simulink model "lab5starter"  (R2022b)
settings: Solver=FixedStepAuto  StartTime=0.0  StopTime=inf  FixedStep=0.002  RelTol=1e-3  EnableMultiTasking=on
undefined symbols (not defined in the file): HIL, Kc, qc_get_step_size, wf, z
libraries: quarc_library x4
settings Model: ExtModeTrigDuration=10000  Creator=lis3  LastModifiedBy=robert
settings SolverCC: PositivePriorityOrder=on
settings DebuggingCC: UnconnectedInputMsg=warning  UnconnectedOutputMsg=warning  UnconnectedLineMsg=warning
settings HardwareCC: ProdBitPerPointer=32  ProdBitPerSizeT=32  ProdBitPerPtrDiffT=32  ProdLargestAtomicInteger=Long  ProdWordSize=32  ProdHWDeviceType=ARM Compatible->ARM 7
settings ModelReferenceCC: EnableRefExpFcnMdlSchedulingChecks=on
settings RTWCC: Description=QUARC Linux RT ARMv7 Target (NI ELVIS III, NI myRIO) Using Toolchain  SystemTargetFile=quarc_linux_rt_armv7.tlc  Toolchain=QUARC linux_rt_armv7 | gmake (64-bit Windows)  BuildConfiguration=Faster Runs  DLArmComputeVersion=19.05
settings STFCustomTargetCC: TargetLangStandard=C99 (ISO)  ConcurrentExecutionCompliant=on  GRTInterface=on  UseToolchainInfoCompliant=on  SystemTargetFile=quarc_linux_rt_armv7.tlc
settings GRTTargetCC: ParMdlRefBuildCompliant=off  CompOptLevelCompliant=off  CombineOutputUpdateFcns=off  MatFileLogging=off  CPPClassGenCompliant=off  GRTInterface=on  ExtMode=on  ExtModeMexFile=quarc_comm  ExtModeMexArgs='-w -d /tmp -uri %u'

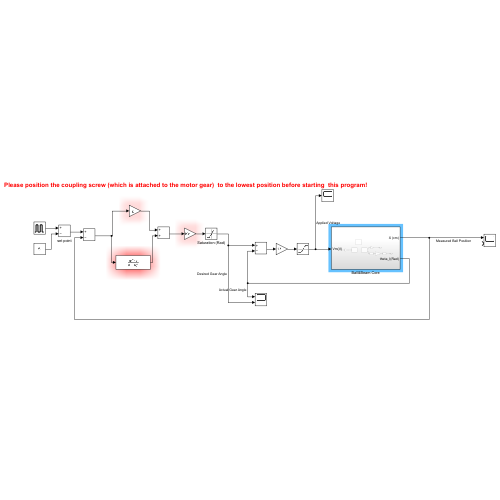
[thumbnail: Simulink's stored preview of the top-level diagram]
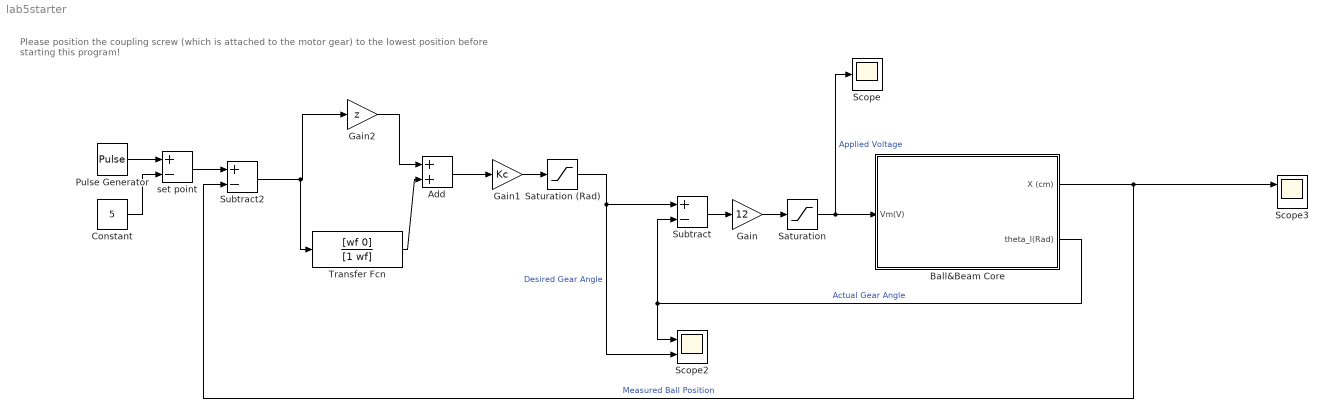
== system lab5starter ==
  note: Please position the coupling screw (which is attached to the motor gear) to the lowest position before starting this program!
  Add : Sum
  Ball&Beam Core : Subsystem
  Constant : Constant  Value=5
  Gain : Gain  Gain=12
  Gain1 : Gain  Gain=Kc
  Gain2 : Gain  Gain=z
  Pulse Generator : DiscretePulseGenerator  PulseType=Time based  Amplitude=10  Period=40  PulseWidth=50
  Saturation : Saturate  UpperLimit=9.5  LowerLimit=-9.5
  Saturation (Rad) : Saturate  UpperLimit=0.942  LowerLimit=-0.942
  Scope : Scope
  Scope2 : Scope  NumInputPorts=2
  Scope3 : Scope  NumInputPorts=2
  Subtract : Sum  Inputs=+-
  Subtract2 : Sum  Inputs=+-
  Transfer Fcn : TransferFcn  Numerator=[wf 0]  Denominator=[1 wf]
  set point : Sum  Inputs=+-
  wires:
  Saturation/1 -> Scope/1, Ball&Beam Core/1(Vm(V))  "Applied Voltage"
  Gain/1 -> Saturation/1
  Subtract/1 -> Gain/1
  Ball&Beam Core/2(theta_I(Rad)) -> Scope2/1, Subtract/2  "Actual Gear Angle"
  Saturation (Rad)/1 -> Subtract/1, Scope2/2  "Desired Gear Angle"
  Gain1/1 -> Saturation (Rad)/1
  Gain2/1 -> Add/1
  Transfer Fcn/1 -> Add/2
  Add/1 -> Gain1/1
  Ball&Beam Core/1(X (cm)) -> Scope3/1, Subtract2/2  "Measured Ball Position"
  Subtract2/1 -> Transfer Fcn/1, Gain2/1
  set point/1 -> Subtract2/1
  Pulse Generator/1 -> set point/1
  Constant/1 -> set point/2

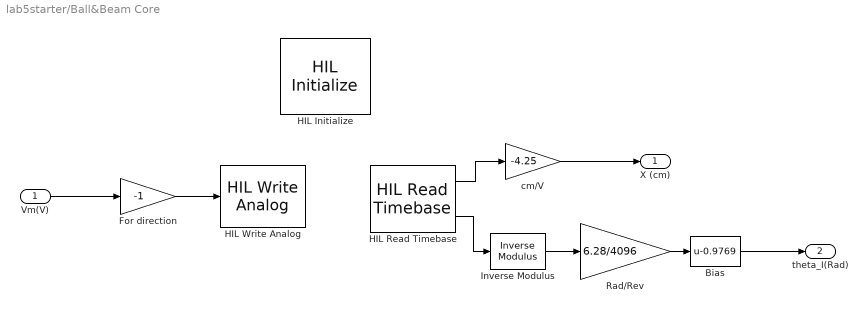
== system lab5starter/Ball&Beam Core ==
  Vm(V) : Inport
  Bias : Bias  Bias=-0.9769  SaturateOnIntegerOverflow=off
  For direction : Gain  Gain=-1
  HIL Initialize : quarc_library/Data Acquisition/Generic/Configuration/HIL Initialize  object_name=HIL-1  board_type=ni_myrio_1900  board_number=0  board_options=enc0_en=1,enc1_en=1,enc2_en=1,enc3_en=1,pwm0_en=1,pwm1_en=1,pwm2_en=1,pwm3_en=1,pwm4_en=1,pwm5_en=1,pwm6_en=1,pwm7_en=1  exclusive=off  active=on  hardware_clocks=[]  clock_modes=[]  initial_clock_frequencies=[]  set_clock_params_at_start=off  set_clock_params_at_switch_in=off  set_clock_frequencies_at_start=off  set_clock_frequencies_at_switch_in=off  analog_input_channels=[0:11]  analog_input_configurations=[]  analog_input_maximums=[5 5 5 5 5 5 5 5 10 10 2.5 2.5]  analog_input_minimums=[0 0 0 0 0 0 0 0 -10 -10 -2.5 -2.5]  set_analog_input_params_at_start=off  set_analog_input_params_at_switch_in=off  analog_output_channels=[0:7]  analog_output_maximums=[5 5 5 5 10 10 2.5 2.5]  analog_output_minimums=[0 0 0 0 -10 -10 -2.5 -2.5]  initial_analog_outputs=[0]  final_analog_outputs=[0]  watchdog_analog_outputs=[]  set_analog_output_params_at_start=off  set_analog_output_params_at_switch_in=off  set_analog_outputs_at_start=on  set_analog_outputs_at_switch_in=off  set_analog_outputs_at_terminate=on  set_analog_outputs_at_switch_out=off  set_analog_outputs_on_watchdog=off  digital_input_channels=[]  digital_output_channels=[]  digital_output_configuration=[]  initial_digital_outputs=[1]  final_digital_outputs=[1]  watchdog_digital_outputs=[]  set_digital_output_params_at_start=off  set_digital_output_params_at_switch_in=off  set_digital_outputs_at_start=on  set_digital_outputs_at_switch_in=off  set_digital_outputs_at_terminate=on  set_digital_outputs_at_switch_out=off  set_digital_outputs_on_watchdog=off  encoder_channels=[2]  quadrature=[4]  encoder_filter_frequency=[]  initial_encoder_counts=[0]  set_encoder_params_at_start=on  set_encoder_params_at_switch_in=off  set_encoder_counts_at_start=on  set_encoder_counts_at_switch_in=off  pwm_channels=[]  pwm_modes=[0]  pwm_frequency=9765.625  pwm_configuration=[]  pwm_alignment=[]  pwm_polarity=[]  pwm_leading_deadband=[]  pwm_trailing_deadband=[]  initial_pwm_outputs=[0]  final_pwm_outputs=[0]  watchdog_pwm_outputs=[]  set_pwm_params_at_start=on  set_pwm_params_at_switch_in=off  set_pwm_outputs_at_start=on  set_pwm_outputs_at_switch_in=off  set_pwm_outputs_at_terminate=on  set_pwm_outputs_at_switch_out=off  set_pwm_outputs_on_watchdog=off  other_output_channels=[]  initial_other_outputs=[]  final_other_outputs=[]  watchdog_other_outputs=[]  set_other_outputs_at_start=off  set_other_outputs_at_switch_in=off  set_other_outputs_at_terminate=off  set_other_outputs_at_switch_out=off  set_other_outputs_on_watchdog=off
  HIL Read Timebase : quarc_library/Data Acquisition/Generic/Timebases/HIL Read Timebase  object_name=HIL-1  clock=0  analog_channels=[9]  encoder_channels=[2]  digital_channels=[]  other_channels=[]  active=on  vector_output=off  data_type_mode=Inherit via back propagation  encoder_data_type=double  digital_data_type=boolean  overflow_mode=Error on overflow  samples_in_buffer=max(ceil(1/qc_get_step_size), 1)
  HIL Write Analog : quarc_library/Data Acquisition/Generic/Immediate I//O/HIL Write Analog  object_name=HIL-1  channels=[4]  sample_time=-1  active=off  vector_input=off
  Inverse Modulus : quarc_library/Discontinuities/Inverse Modulus  modulus=2^32  output_derivative=off  output_revolutions=off  max_x=Inf  min_x=-Inf
  Rad/Rev : Gain  Gain=6.28/4096
  cm/V : Gain  Gain=-4.25
  X (cm) : Outport
  theta_I(Rad) : Outport  Port=2
  wires:
  Vm(V)/1 -> For direction/1
  Bias/1 -> theta_I(Rad)/1
  HIL Read Timebase/2 -> Inverse Modulus/1
  HIL Read Timebase/1 -> cm/V/1
  For direction/1 -> HIL Write Analog/1
  Inverse Modulus/1 -> Rad/Rev/1
  Rad/Rev/1 -> Bias/1
  cm/V/1 -> X (cm)/1
